simulink model "tanque_simulink"  (R2019b)
settings: Solver=VariableStepAuto  StartTime=0.0  StopTime=200.0  RelTol=1e-3
values from neighbouring files (symbols this model uses):
  ang = pi/3    (= 1.0471975512)    [tanque_simulink_param.m]
  g = 9.8    [tanque_simulink_param.m]
  h_ini = 0.6    [tanque_simulink_param.m]
  p_apertura = 1    [tanque_simulink_param.m]
  Q_ent = 0.0035    [tanque_simulink_param.m]
  r_apertura = 0.0254    [tanque_simulink_param.m]
  rad_menor = 0.05    [tanque_simulink_param.m]
settings Model: Creator=Franco  LastModifiedBy=Franco

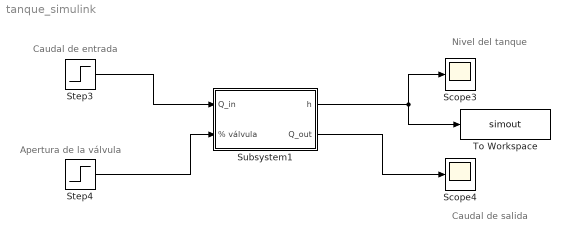
== system tanque_simulink ==
  note: Caudal de salida
  note: Nivel del tanque
  note: Apertura de la válvula
  note: Caudal de entrada
  Scope3 : Scope
  Scope4 : Scope
  Step3 : Step  After=Q_ent  SampleTime=0
  Step4 : Step  After=p_apertura  SampleTime=0
  Subsystem1 : Subsystem
  To Workspace : ToWorkspace  VariableName=simout  SaveFormat=Timeseries  SampleTime=-1
  wires:
  Step3/1 -> Subsystem1/1(Q_in)
  Subsystem1/2(Q_out) -> Scope4/1
  Subsystem1/1(h) -> To Workspace/1, Scope3/1
  Step4/1 -> Subsystem1/2(" % válvula")

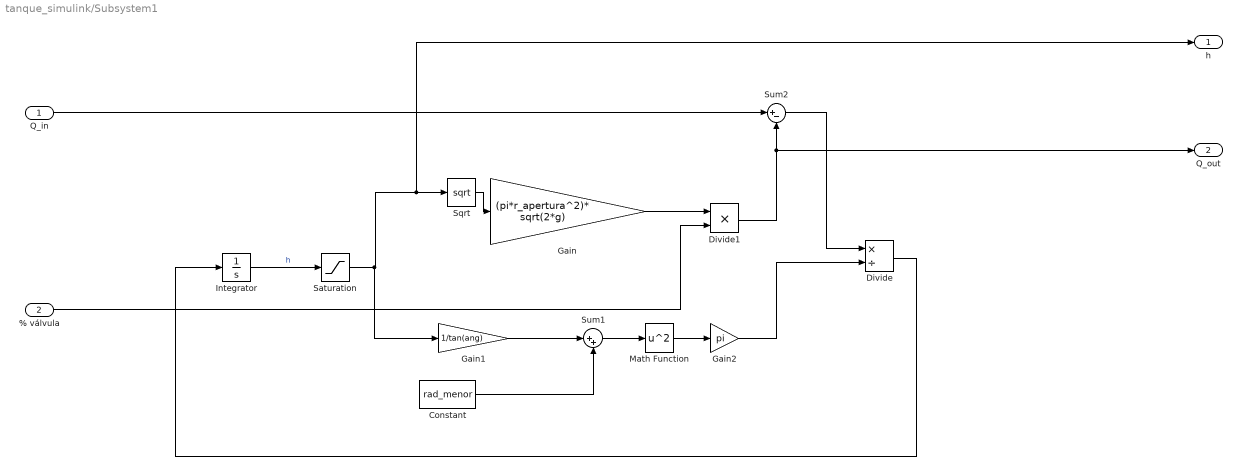
== system tanque_simulink/Subsystem1 ==
  Q_in : Inport
  " % válvula" : Inport  Port=2
  Constant : Constant  Value=rad_menor
  Divide : Product  Inputs=*/
  Divide1 : Product  Inputs=**
  Gain : Gain  Gain=(pi*r_apertura^2)* sqrt(2*g)
  Gain1 : Gain  Gain=1/tan(ang)
  Gain2 : Gain  Gain=pi
  Integrator : Integrator  InitialCondition=h_ini
  Math Function : Math  Operator=square  SignedPower=off  SaturateOnIntegerOverflow=on
  Saturation : Saturate  UpperLimit=1  LowerLimit=0
  Sqrt : Sqrt  SaturateOnIntegerOverflow=on
  Sum1 : Sum  Inputs=|++
  Sum2 : Sum  Inputs=|+-
  h : Outport
  Q_out : Outport  Port=2
  wires:
  Gain/1 -> Divide1/1
  Integrator/1 -> Saturation/1  "h"
  Sqrt/1 -> Gain/1
  Sum2/1 -> Divide/1
  Math Function/1 -> Gain2/1
  Saturation/1 -> Gain1/1, h/1, Sqrt/1
  Gain1/1 -> Sum1/1
  Sum1/1 -> Math Function/1
  Divide/1 -> Integrator/1
  Gain2/1 -> Divide/2
  Q_in/1 -> Sum2/1
  Constant/1 -> Sum1/2
  " % válvula"/1 -> Divide1/2
  Divide1/1 -> Q_out/1, Sum2/2
